simulink model "MPC_experimental_uncontrolled"  (Simulink 7.6)
settings: Solver=ode3  StartTime=0.0  StopTime=inf  FixedStep=.05  RelTol=1e-3
InitFcn:
  | a2g = 1/9.81;
  | r2d = 180/pi;
  | K_sr = 15.97;
  | neutral_steer = 103;
  | s2t = (pi/180)*(1/K_sr);
  | A_kt =[         0         0         0         0         0         0
  |          0   -3.5058   -1.6990  -25.6114   -2.2435         0
  |          0    2.2782   -4.2575  -64.1772   -5.6218         0
  |          0         0    1.0000         0         0         0
  |          0   -0.0158    0.0295    0.4442   -4.1900         0
  |          0         0         0         0    1.0000         0];
  | 
  | 
  | B_kt =[0
  |    23.7845
  |   -16.0342
  |          0
  |    17.5770
  |          0];
  | 
  | load MPC_test_2
StopFcn:
  | %x = x_values.signals.values;
  | %y = -y_values.signals.values;
  | %yL = y + 0.5;
  | %yR = y - 0.5;
  | 
  | %hold all;
  | 
  | %plot(x,yL,'r');
  | %plot(x,yR,'r');
  | 
  | %line([15 17],[0 0]);
  | %line([15 17],[-1 -1]);
  | %line([15 15],[0 -1]);
  | %line([17 17],[0 -1]);
  | %axis([0 30 -5 5]);
  | 
  | %hold off;
undefined symbols (not defined in the file or in its folder): CR, DiscIntNeverNeededParam, serial
libraries: instrumentlib x3, dspadpt3 x1, realtime_pacer_lib x1
settings Model: Creator=TCA  LastModifiedBy=ipainter  BufferReuse=off
settings OptimizationCC: BlockReduction=off  InlineParams=on  BufferReuse=off  InitFltsAndDblsToZero=on
settings DebuggingCC: AlgebraicLoopMsg=none  SolverPrmCheckMsg=none  InheritedTsInSrcMsg=none  UnconnectedInputMsg=none  UnconnectedOutputMsg=none  UnconnectedLineMsg=none  StrictBusMsg=Warning
settings SFSimCC: SimParseCustomCode=off

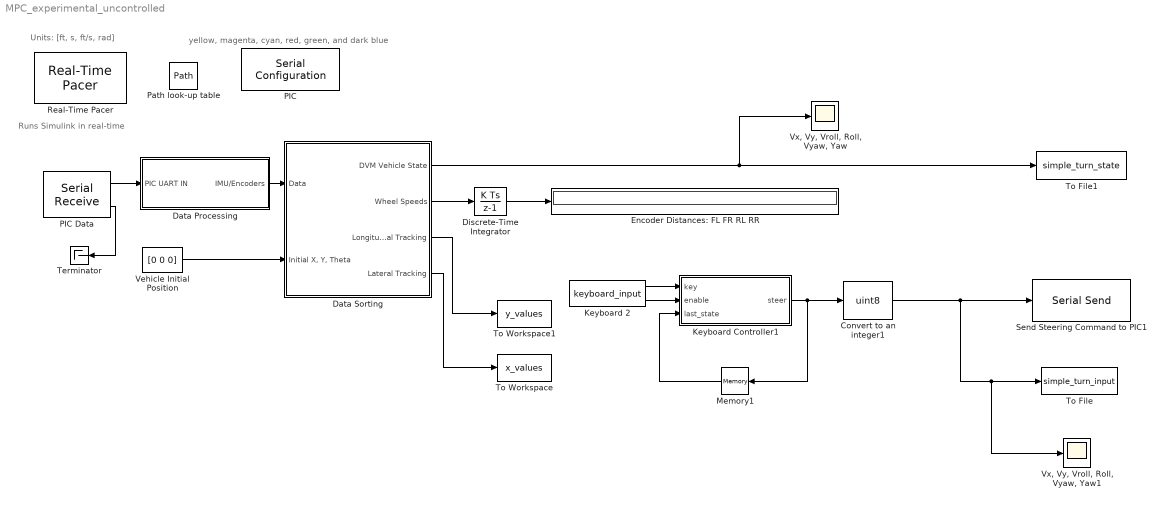
== system MPC_experimental_uncontrolled ==
  note: Runs Simulink
      |  in real-time
  note: Units: [ft, s, ft/s, rad]
  note: yellow, magenta, cyan, red, green, and dark blue
  Convert to an integer1 : DataTypeConversion  OutDataTypeStr=uint8  SampleTime=.05  SaturateOnIntegerOverflow=on  RndMeth=Zero
  Data Processing : Subsystem
  Data Sorting : Subsystem
  Discrete-Time Integrator : DiscreteIntegrator  SampleTime=0.05  ICPrevOutput=DiscIntNeverNeededParam  ICPrevScaledInput=DiscIntNeverNeededParam
  Encoder Distances: FL FR RL RR : Display
  Keyboard Controller1 : Stateflow chart  TreatAsAtomicUnit=on
  Keyboard 2 : M-S-Function  FunctionName=keyboard_input
      mask Type: Keyboard Input
      mask Description: Keyboard Input
      mask Display: fprintf('Keyboard');
  Memory1 : Memory  X0=[250,103,120]  InheritSampleTime=on
  PIC : instrumentlib/Serial Configuration  Priority=-200000  DialogController=instrumentcreatedialog  DialogControllerArgs=DataTag1  ComPortMenu=COM5  ComPort=COM5  ObjConstructor=serial('COM5');  BaudRate=9600  DataBits=8  Parity=none  StopBits=1  FlowControl=none  Timeout=10  ByteOrder=LittleEndian
  PIC Data : instrumentlib/Serial Receive  DialogController=instrumentcreatedialog  DialogControllerArgs=DataTag2  ComPortMenu=COM5  ComPort=COM5  ObjConstructor=serial('COM5');  Terminator=CR ('\r')  DataSize="[1  16]"  DataType=uint8  EnableBlockingMode=off  ActionDataUnavailable=Output last received value  CustomValue=0  SampleTime=.05
  Path look-up table : DataStoreMemory  DataStoreName=Path  ReadBeforeWriteMsg=warning  WriteAfterWriteMsg=warning  WriteAfterReadMsg=warning  InitialValue=zeros(50, 6)  VectorParams1D=off
  Real-Time Pacer : realtime_pacer_lib/Real-Time Pacer  simTimePerRealTime=1
  Send Steering Command to PIC1 : instrumentlib/Serial Send  DialogController=instrumentcreatedialog  DialogControllerArgs=DataTag3  ComPortMenu=COM5  ComPort=COM5  ObjConstructor=serial('COM5');  Header=250  Terminator=<none>  EnableBlockingMode=off
  Terminator : Terminator
  To File : ToFile  Filename=simple_turn_input  MatrixName=ST_input  SaveFormat=Timeseries
  To File1 : ToFile  Filename=simple_turn_state  MatrixName=ST_state  SaveFormat=Timeseries
  To Workspace : ToWorkspace  VariableName=x_values  SampleTime=-1  SaveFormat=Structure
  To Workspace1 : ToWorkspace  VariableName=y_values  SampleTime=-1  SaveFormat=Structure
  Vehicle Initial Position : Constant  Value=[0 0 0]  VectorParams1D=off
  "Vx, Vy, Vroll, Roll, Vyaw, Yaw" : Scope
      settings: TimeRange=10  YMax=30  SaveName=ScopeData2
  "Vx, Vy, Vroll, Roll, Vyaw, Yaw1" : Scope
      settings: TimeRange=10  YMax=30
  wires:
  PIC Data/2 -> Terminator/1
  Vehicle Initial Position/1 -> Data Sorting/2("Initial X, Y, Theta")
  PIC Data/1 -> Data Processing/1(PIC UART IN)
  Data Processing/1(IMU/Encoders) -> Data Sorting/1(Data)
  Discrete-Time Integrator/1 -> Encoder Distances: FL FR RL RR/1
  Data Sorting/2(Wheel Speeds) -> Discrete-Time Integrator/1
  Data Sorting/3(Longitudinal Tracking) -> To Workspace1/1
  Data Sorting/4(Lateral Tracking) -> To Workspace/1
  Data Sorting/1(DVM Vehicle State) -> "Vx, Vy, Vroll, Roll, Vyaw, Yaw"/1, To File1/1
  Keyboard Controller1/1(steer) -> Convert to an integer1/1, Memory1/1
  Memory1/1 -> Keyboard Controller1/3(last_state)
  Keyboard 2/1 -> Keyboard Controller1/1(key)
  Keyboard 2/2 -> Keyboard Controller1/2(enable)
  Convert to an integer1/1 -> Send Steering Command to PIC1/1, To File/1, "Vx, Vy, Vroll, Roll, Vyaw, Yaw1"/1

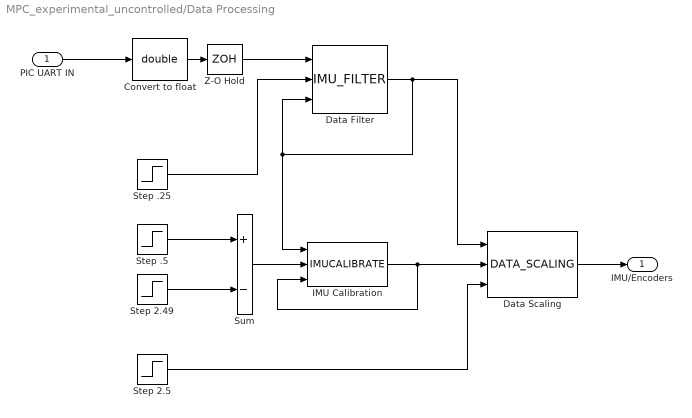
== system MPC_experimental_uncontrolled/Data Processing ==
  PIC UART IN : Inport
  Convert to float : DataTypeConversion  OutDataTypeStr=double  SaturateOnIntegerOverflow=on  RndMeth=Zero
  Data Filter : M-S-Function  FunctionName=IMU_FILTER  Parameters=3
  "Data Scaling " : M-S-Function  FunctionName=DATA_SCALING  Parameters=3
  IMU Calibration : M-S-Function  FunctionName=IMUCALIBRATE  Parameters=3
  Step .25 : Step  Time=.25  SampleTime=0
  Step .5 : Step  Time=.5  SampleTime=0
  Step 2.49 : Step  Time=2.49  SampleTime=0
  Step 2.5 : Step  Time=2.5  SampleTime=0
  Sum : Sum  Inputs=+-
  Z-O Hold : ZeroOrderHold  SampleTime=0.05
  IMU/Encoders : Outport
  wires:
  Convert to float/1 -> Z-O Hold/1
  Data Filter/1 -> "Data Scaling "/1, IMU Calibration/1, Data Filter/3
  IMU Calibration/1 -> IMU Calibration/3, "Data Scaling "/2
  Step .5/1 -> Sum/1
  Step 2.49/1 -> Sum/2
  Z-O Hold/1 -> Data Filter/1
  Step .25/1 -> Data Filter/2
  Sum/1 -> IMU Calibration/2
  Step 2.5/1 -> "Data Scaling "/3
  "Data Scaling "/1 -> IMU/Encoders/1
  PIC UART IN/1 -> Convert to float/1

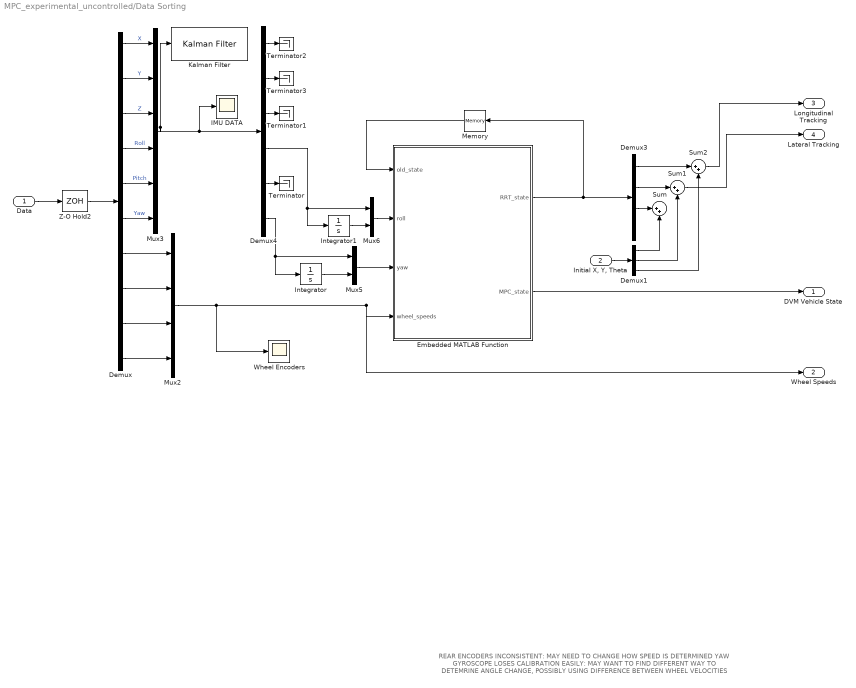
== system MPC_experimental_uncontrolled/Data Sorting ==
  note: REAR ENCODERS INCONSISTENT: MAY NEED TO CHANGE HOW SPEED IS DETERMINED
      | YAW GYROSCOPE LOSES CALIBRATION EASILY: MAY WANT TO FIND DIFFERENT WAY TO DETEMRINE
      | ANGLE CHANGE, POSSIBLY USING DIFFERENCE BETWEEN WHEEL VELOCITIES
  Data : Inport
  "Initial X, Y, Theta" : Inport  Port=2
  Demux : Demux  Outputs=10
  Demux1 : Demux  Outputs=3
  Demux3 : Demux
  Demux4 : Demux  Outputs=6
  Embedded MATLAB Function : Stateflow chart  TreatAsAtomicUnit=on
  IMU DATA : Scope
      settings: SaveName=ScopeData3
  Integrator : Integrator
  Integrator1 : Integrator
  Kalman Filter : dspadpt3/Kalman Filter  DialogController=dspDDGCreate  DialogControllerArgs=DataTag0  SystemSampleTime=-1  num_targets=1  sourceEnable=Always  isReset=on  X=zeros(6,1)  P=10*eye(6)  A=eye(6)  sourceMeasure=Specify via Dialog  H=eye(6)  Q=0.05*eye(6)  R=eye(6)  isOutputEstMeasure=on  isOutputEstState=off  isOutputEstError=off  isOutputPrdMeasure=off  isOutputPrdState=off  isOutputPrdError=off
  Memory : Memory  X0=[0,0,0,0]  InheritSampleTime=on
  Mux2 : Mux
  Mux3 : Mux  Inputs=6
  Mux5 : Mux  Inputs=2
  Mux6 : Mux  Inputs=2
  Sum : Sum  Inputs=|++
  Sum1 : Sum  Inputs=|++
  Sum2 : Sum  Inputs=|++
  Terminator{,1..3} (4 alike) : Terminator
  Wheel Encoders : Scope
  Z-O Hold2 : ZeroOrderHold  SampleTime=0.05
  DVM Vehicle State : Outport
  Wheel Speeds : Outport  Port=2
  Longitudinal Tracking : Outport  Port=3
  Lateral Tracking : Outport  Port=4
  wires:
  Data/1 -> Z-O Hold2/1
  "Initial X, Y, Theta"/1 -> Demux1/1
  Memory/1 -> Embedded MATLAB Function/1(old_state)
  Embedded MATLAB Function/1(RRT_state) -> Memory/1, Demux3/1
  Demux/6 -> Mux3/6  "Yaw"
  Demux/1 -> Mux3/1  "X"
  Demux/2 -> Mux3/2  "Y"
  Mux3/1 -> Kalman Filter/1, Demux4/1, IMU DATA/1
  Demux/3 -> Mux3/3  "Z"
  Demux/4 -> Mux3/4  "Roll"
  Demux/5 -> Mux3/5  "Pitch"
  Demux/7 -> Mux2/1
  Demux/8 -> Mux2/2
  Demux/9 -> Mux2/3
  Demux/10 -> Mux2/4
  Mux2/1 -> Embedded MATLAB Function/4(wheel_speeds), Wheel Speeds/1, Wheel Encoders/1
  Z-O Hold2/1 -> Demux/1
  Demux1/1 -> Sum/2
  Demux1/2 -> Sum1/2
  Demux1/3 -> Sum2/2
  Demux3/2 -> Sum1/1
  Demux3/1 -> Sum2/1
  Demux3/3 -> Sum/1
  Sum2/1 -> Longitudinal Tracking/1
  Sum1/1 -> Lateral Tracking/1
  Demux4/4 -> Integrator1/1, Mux6/1
  Demux4/6 -> Integrator/1, Mux5/1
  Integrator/1 -> Mux5/2
  Mux5/1 -> Embedded MATLAB Function/3(yaw)
  Integrator1/1 -> Mux6/2
  Mux6/1 -> Embedded MATLAB Function/2(roll)
  Demux4/5 -> Terminator/1
  Demux4/3 -> Terminator1/1
  Demux4/1 -> Terminator2/1
  Demux4/2 -> Terminator3/1
  Embedded MATLAB Function/2(MPC_state) -> DVM Vehicle State/1

== matlab function Data Sorting/Embedded MATLAB Function ==
  data: old_state input double; roll input double; yaw input double; wheel_speeds input double; RRT_state output double; MPC_state output double
% function [x,y,theta,velocity, TESTING] = fcn(x_old,y_old,theta_old,yaw_rate_IMU,Vl_old,Vr_old)
% %#eml
% 
% deltaK = 0.05;
% 
% delta_theta_enc = (Vr_old - Vl_old)*(12/10)*deltaK;
% delta_theta_imu = yaw_rate_IMU*deltaK;
% delta_theta = (delta_theta_enc+delta_theta_imu)/2;
% 
% theta = theta_old + delta_theta;
% 
% velocity = (Vl_old + Vr_old)/2;
% 
% x = x_old + velocity*-1*sin(theta_old)*deltaK;
% y = y_old + velocity*cos(theta_old)*deltaK;

%NEW AWESOME DATA SORTING
function [RRT_state,MPC_state]  = data_sorting(old_state,roll,yaw, wheel_speeds)
%#eml
deltaK = 0.05;

x_old = old_state(1);
y_old = old_state(2);

velocity = (wheel_speeds(1) + wheel_speeds(2) + wheel_speeds(3) + wheel_speeds(4))/4;

Phi_d = roll(1);
Phi = roll(2);
Psi_d = yaw(1);
Psi = yaw(2);
Vx = velocity*sin(Psi);
Vy = velocity*cos(Psi); 

x = x_old - Vx*deltaK;
y = y_old + Vy*deltaK;

MPC_state = [Vx*(1/3.28), Vy*(1/3.28), Phi_d, Phi, Psi_d, Psi]';
RRT_state = [x, y, Psi, velocity]';

== matlab function Keyboard Controller1 ==
  data: key input double; enable input double; steer output double; last_state input double
function steer = key_to_steer(key,enable,last_state)
%#eml
steer = last_state;

switch key

    case 28        %right
        steer(2) = 5;
    
    case 29        %left
        steer(2) = 235;
    
    case 30        %forward
        steer(2) = 100;
        steer(3) = 200;
    
    case 31        %stop/reverse
        steer(2) = 100;
        steer(3) = 100;
end

% if enable
%     switch key
% 
%         case 28        %right
%             steer(2) = steer(2) - 10;
% 
%         case 29        %left
%             steer(2) = steer(2) + 10;
%     end
% end
